simulink library "timer_lib"  (Simulink 6.6)
libraries: simulink x1, timer_lib x1
settings Model: Creator=Austin Murch  LastModifiedBy=cox  ExtModeAutoUpdateStatusClock=off

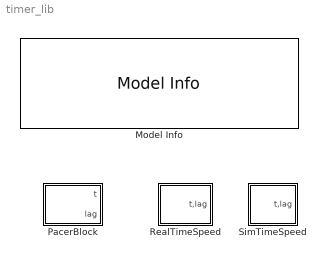
== system timer_lib ==
  Model Info : simulink/Model-Wide Utilities/Model Info  SystemSampleTime=-1  InitialBlockCM=None  BlockCM=None  Frame=on  DisplayStringWithTags=|  HorizontalTextAlignment=Center  LeftAlignmentValue=0.5  SourceBlockDiagram=timer_lib  TagMaxNumber=20
      | Timer Library
      | %<ModelVersion>
      | Las modified by %<LastModifiedBy> on %<LastModificationDate>
  PacerBlock : Subsystem  BlockChoice=RealTimeSpeed
      settings: TemplateBlock=self  MemberBlocks=RealTimeSpeed,SimTimeSpeed
  RealTimeSpeed : Subsystem
  SimTimeSpeed : Subsystem

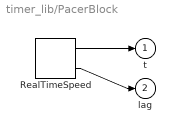
== system timer_lib/PacerBlock ==
  RealTimeSpeed : timer_lib/RealTimeSpeed  SystemSampleTime=-1
  t : Outport
  lag : Outport  Port=2
  wires:
  RealTimeSpeed/1 -> t/1
  RealTimeSpeed/2 -> lag/1

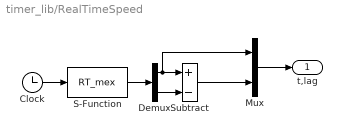
== system timer_lib/RealTimeSpeed ==
  Clock : Clock
      settings: Decimation=10
  Demux : Demux  Outputs=2
  Mux : Mux  Inputs=2
  S-Function : S-Function  FunctionName=RT_mex
  Subtract : Sum  Inputs=+-  OutScaling=2^-10
  t,lag : Outport
  wires:
  Clock/1 -> S-Function/1
  S-Function/1 -> Demux/1
  Demux/1 -> Subtract/1, Mux/1
  Demux/2 -> Subtract/2
  Subtract/1 -> Mux/2
  Mux/1 -> t,lag/1

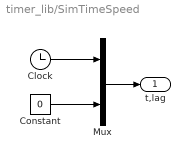
== system timer_lib/SimTimeSpeed ==
  Clock : Clock
      settings: Decimation=10
  Constant : Constant  Value=0
  Mux : Mux  Inputs=2
  t,lag : Outport
  wires:
  Clock/1 -> Mux/1
  Constant/1 -> Mux/2
  Mux/1 -> t,lag/1
